simulink model "W03_S1"  (R2024b)
settings: Solver=ode4  StartTime=0  StopTime=T_final  FixedStep=h  RelTol=1e-3
values from neighbouring files (symbols this model uses):
  Kp = logspace(1.5, 4, 60)    [W03_S_expected.m]
undefined symbols (not defined in the file or in its folder): beta_c, DiscIntNeverNeededParam, h, Ki, loop_closed, mp, rp, t_step, u_d, V_c, x0, X_open
settings Model: Creator=admin  LastModifiedBy=admin
settings DataIOCC: ReturnWorkspaceOutputs=off

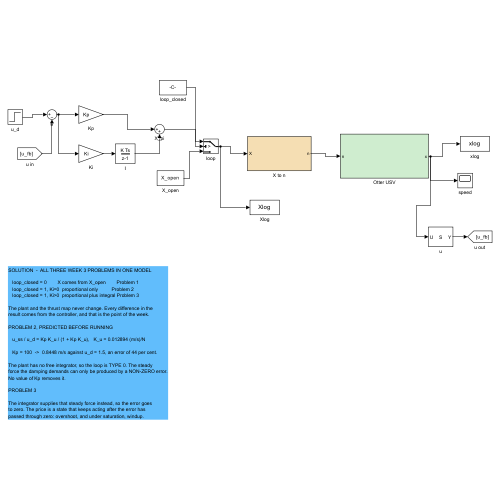
[thumbnail: Simulink's stored preview of the top-level diagram]
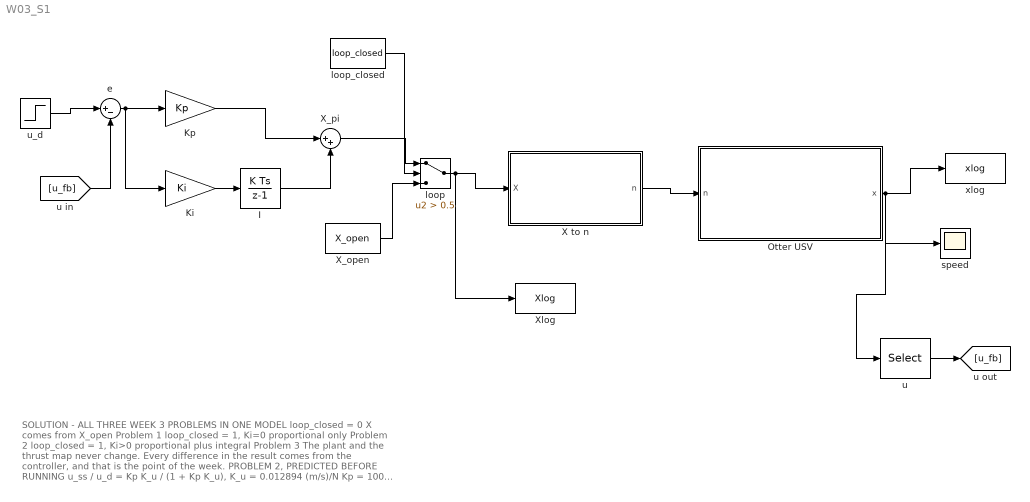
== system W03_S1 ==
  note: SOLUTION  -  ALL THREE WEEK 3 PROBLEMS IN ONE MODEL
      |
      |    loop_closed = 0        X comes from X_open        Problem 1
      |    loop_closed = 1, Ki=0  proportional only          Problem 2
      |    loop_closed = 1, Ki>0  proportional plus integral Problem 3
      |
      | The plant and the thrust map never change. Every difference in the
      | result comes from the controller, and that is the point of the week.
      |
      | PROBLEM 2, PREDICTED BEFORE RUNNING
      |
      |    u_ss / u_d = Kp K_u / (1 + Kp K_u),   K_u = 0.012894 (m/s)/N
      |
      |    Kp = 100  ->  0.8448 m/s against u_d = 1.5, an error of 44 per cent.
      |
      | The plant has no free integrator, so the loop is TYPE 0. The steady
      | force the damping demands can only be produced by a NON-ZERO error.
      | No value of Kp removes it.
      |
      | PROBLEM 3
      |
      | The integrator supplies that steady force instead, so the error goes
      | to zero. The price is a state that keeps acting after the error has
      | passed through zero: overshoot, and under saturation, windup.
  I : DiscreteIntegrator  SampleTime=h  ICPrevOutput=DiscIntNeverNeededParam  ICPrevScaledInput=DiscIntNeverNeededParam
  Ki : Gain  Gain=Ki
  Kp : Gain  Gain=Kp
  Otter USV : Subsystem
  X to n : Subsystem
  X_open : Constant  Value=X_open
  X_pi : Sum  Inputs=|++
  Xlog : ToWorkspace  VariableName=Xlog  SaveFormat=Structure With Time  SampleTime=-1
  e : Sum  Inputs=|+-
  loop : Switch  Criteria=u2 > Threshold  Threshold=0.5  SaturateOnIntegerOverflow=off  InputSameDT=off
  loop_closed : Constant  Value=loop_closed
  speed : Scope
  u : Selector  InputPortWidth=12  IndexOptions=Index vector (dialog)  Indices=1  OutputSizes=1
  u_d : Step  Time=t_step  After=u_d  SampleTime=0
  xlog : ToWorkspace  VariableName=xlog  SaveFormat=Structure With Time  SampleTime=-1
  wires:
  u_d/1 -> e/1
  e/1 -> Kp/1, Ki/1
  Ki/1 -> I/1
  Kp/1 -> X_pi/1
  I/1 -> X_pi/2
  X_pi/1 -> loop/1
  loop_closed/1 -> loop/2
  X_open/1 -> loop/3
  loop/1 -> X to n/1(X), Xlog/1
  X to n/1(n) -> Otter USV/1(n)
  Otter USV/1(x) -> xlog/1, u/1, speed/1
  u/1 -> [u_fb]
  [u_fb] -> e/2

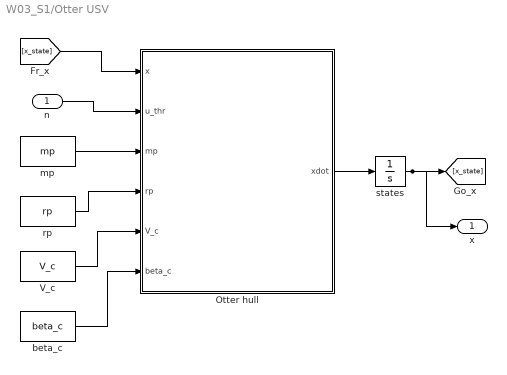
== system W03_S1/Otter USV ==
  n : Inport
  Otter hull : MATLAB Function  TreatAsAtomicUnit=on
  V_c : Constant  Value=V_c
  beta_c : Constant  Value=beta_c
  mp : Constant  Value=mp
  rp : Constant  Value=rp
  states : Integrator  InitialCondition=x0
  x : Outport
  wires:
  mp/1 -> Otter hull/3(mp)
  [x_state] -> Otter hull/1(x)
  n/1 -> Otter hull/2(u_thr)
  rp/1 -> Otter hull/4(rp)
  V_c/1 -> Otter hull/5(V_c)
  Otter hull/1(xdot) -> states/1
  beta_c/1 -> Otter hull/6(beta_c)
  states/1 -> [x_state], x/1

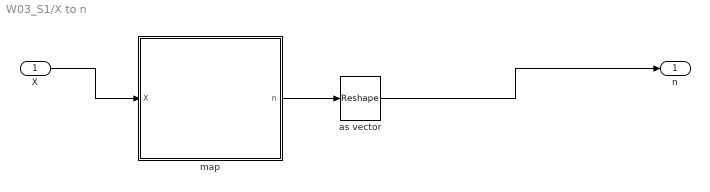
== system W03_S1/X to n ==
  X : Inport
  as vector : Reshape
  map : MATLAB Function  TreatAsAtomicUnit=on
  n : Outport
  wires:
  X/1 -> map/1(X)
  map/1(n) -> as vector/1
  as vector/1 -> n/1

== matlab function W03_S1/Otter USV/Otter hull ==
  data: x input; xdot output double size=[12 1]; u_thr input; mp input; rp input; V_c input; beta_c input
function xdot = otter_hull(x, u_thr, mp, rp, V_c, beta_c)
% Fossen's otter.m, called unchanged from Tools/MSS/VESSELS.
%
%   x       12 states, fed back from the integrator
%   u_thr   propeller shaft speeds [rad/s]
%
% otter.m is not written for code generation, so the call is extrinsic and
% xdot has to be pre-sized for Simulink to know the output width.
coder.extrinsic('otter');

xdot = zeros(12,1);
xdot = otter(x, u_thr, mp, rp, V_c, beta_c);
end

== matlab function W03_S1/X to n/map ==
  data: X input; n output double size=[2 1]
function n = map(X)
%#codegen
%MAP  Demanded surge force -> two equal shaft speeds. Appendix A1 section C.
k_pos = 0.02216/2;   k_neg = 0.01289/2;
n_max =  sqrt((0.5*24.4*9.81)/k_pos);
n_min = -sqrt((0.5*13.6*9.81)/k_neg);
T = X/2;
if T >= 0
    ni =  sqrt(  T  / k_pos);
else
    ni = -sqrt( -T  / k_neg);
end
ni = min(max(ni, n_min), n_max);
n  = [ni; ni];
